simulink model "Ex03"  (R2021b)
settings: Solver=VariableStepAuto  StartTime=0.0  StopTime=3  RelTol=1e-3
settings Model: Creator=carlo  LastModifiedBy=carlo
settings SolverCC: AlgebraicLoopSolver=TrustRegion
settings DebuggingCC: SFMachineParentedDataDiag=warning

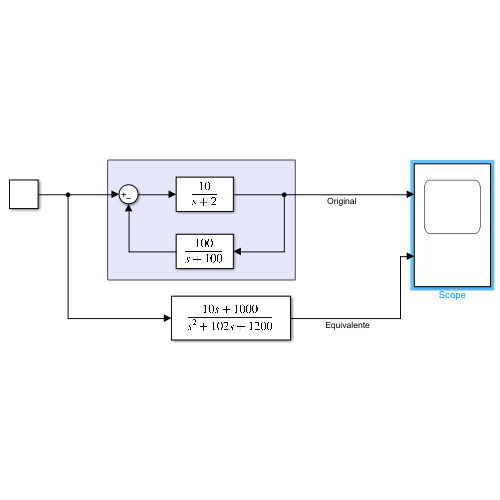
[thumbnail: Simulink's stored preview of the top-level diagram]
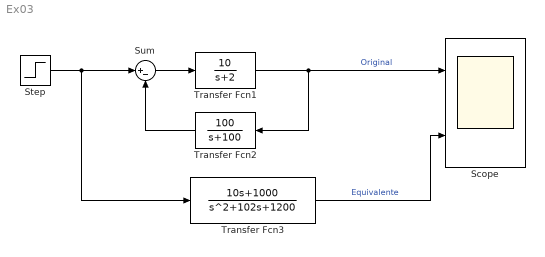
== system Ex03 ==
  Scope : Scope  NumInputPorts=2
  Step : Step  SampleTime=0
  Sum : Sum  Inputs=|+-
  Transfer Fcn1 : TransferFcn  Numerator=[10]  Denominator=[1 2]
  Transfer Fcn2 : TransferFcn  Numerator=[100]  Denominator=[1 100]
  Transfer Fcn3 : TransferFcn  Numerator=[10 1000]  Denominator=[1 102 1200]
  wires:
  Transfer Fcn3/1 -> Scope/2  "Equivalente"
  Step/1 -> Sum/1, Transfer Fcn3/1
  Transfer Fcn2/1 -> Sum/2
  Transfer Fcn1/1 -> Transfer Fcn2/1, Scope/1  "Original"
  Sum/1 -> Transfer Fcn1/1
